simulink model "simusoonnlaan"  (R2021a)
settings: Solver=VariableStepAuto  StartTime=0.0  StopTime=95  RelTol=1e-3
settings Model: Creator=user  LastModifiedBy=Ahmet Talha
settings SolverCC: AlgebraicLoopSolver=TrustRegion
settings DebuggingCC: SFMachineParentedDataDiag=warning

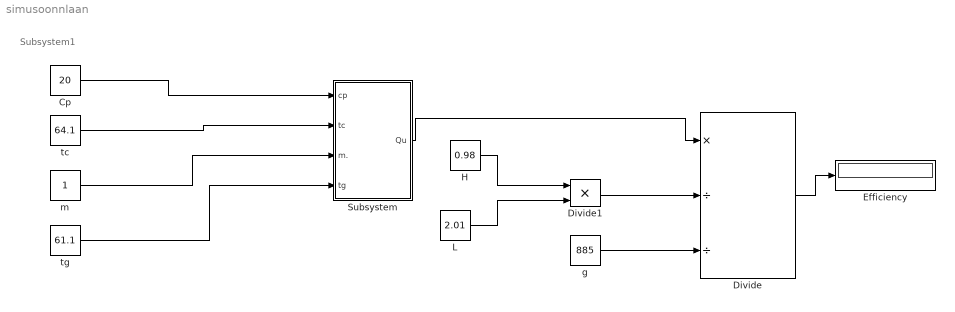
== system simusoonnlaan ==
  note: Subsystem1
  Cp : Constant  Value=20
  Divide : Product  Inputs=*//
  Divide1 : Product  Inputs=**
  Efficiency : Display
  H : Constant  Value=0.98
  L : Constant  Value=2.01
  Subsystem : Subsystem
      mask Display: image('C:\Users\Ahmet Talha\Desktop\matlab projem\solar-photovoltaic-panel-500x500.jpg'); % Use "Edit Image" on toolstrip to change.
  g : Constant  Value=885
  m : Constant
  tc : Constant  Value=64.1
  tg : Constant  Value=61.1
  wires:
  Divide1/1 -> Divide/2
  L/1 -> Divide1/2
  H/1 -> Divide1/1
  tc/1 -> Subsystem/2(tc)
  Cp/1 -> Subsystem/1(cp)
  g/1 -> Divide/3
  tg/1 -> Subsystem/4(tg)
  Subsystem/1(Qu) -> Divide/1
  m/1 -> Subsystem/3(m.)
  Divide/1 -> Efficiency/1

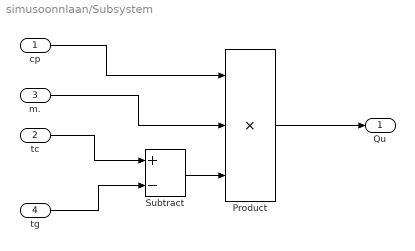
== system simusoonnlaan/Subsystem ==
  cp : Inport
  tc : Inport  Port=2
  m. : Inport  Port=3
  tg : Inport  Port=4
  Product : Product  Inputs=3
  Subtract : Sum  Inputs=+-
  Qu : Outport
  wires:
  cp/1 -> Product/1
  tc/1 -> Subtract/1
  Product/1 -> Qu/1
  Subtract/1 -> Product/3
  tg/1 -> Subtract/2
  m./1 -> Product/2
